simulink model "AdaptiveControlsProjectPart2_Sethi"  (R2019b)
settings: Solver=ode45  StartTime=0.0  StopTime=40  RelTol=1e-6
undefined symbols (not defined in the file): Ar, Astar, B, Br, Bstar, cur0, Gam, Gam_r, Gam_x, J, K, L, Lambda, lambda_star, linp, om0, P, phi0, Q, R, theta0, Tr_star, Tx_star, V0, w10, w20, Xr0
libraries: simulink x1
settings Model: Creator=aleon  LastModifiedBy=Japnit Sethi
settings SFSimCC: CustomCodeUndefinedFunction=UseInterfaceOnly

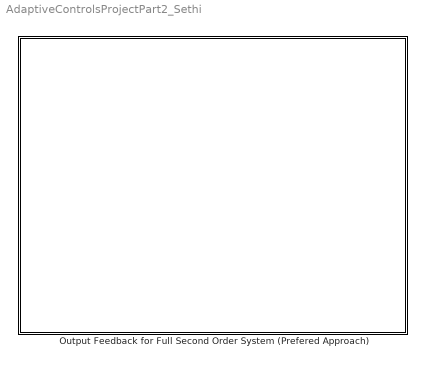
== system AdaptiveControlsProjectPart2_Sethi ==
  Output Feedback for Full Second Order System (Prefered Approach) : Subsystem

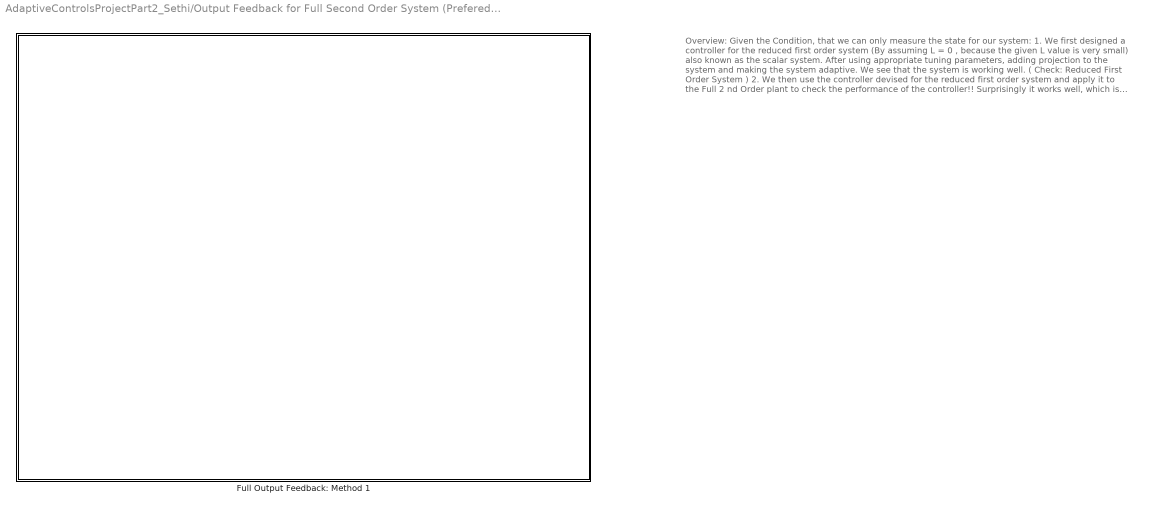
== system AdaptiveControlsProjectPart2_Sethi/Output Feedback for Full Second Order System (Prefered Approach) ==
  note: Overview:
      | Given the Condition, that we can only measure the state for our system:
      | 1. We first designed a controller for the reduced first order system (By assuming L = 0 , because the given L value is very small) also known as the scalar system. After using appropriate tuning parameters, adding projection to the system and making the system adaptive. We see that the system is working well. ( Check: Reduced First Order System )
      | 2. We then use the controller devised for the reduced first order system and apply it to the Full 2 nd Order plant to check the performance of the controller!! Surprisingly it works well, which is because the approximation of L was legible.
      | 3. We designed a Full state feedback controller for the Full second order system, by deriving the equations in canonical form and also change our states from and to and which is important in order to derive and satisfy our compatibility equations. In this scenario, we were able to measure both and . ( Check: Full Second Order System )
      | 4. Finally, we designed a Full Output Feedback controller , because in really, we cannot measure , the only measurement available to us is .
      | Note: ( Option 2: But not recommended ) For the Full output feedback controller above, we could measure and then calculate the by computing a numerical derivative of measured and adding a filter transfer function to get rid of the noise. But this is not preferred because excessive time that we can lose tuning our parameters to get rid of high oscillations and noise.
  Full Output Feedback: Method 1 : Subsystem

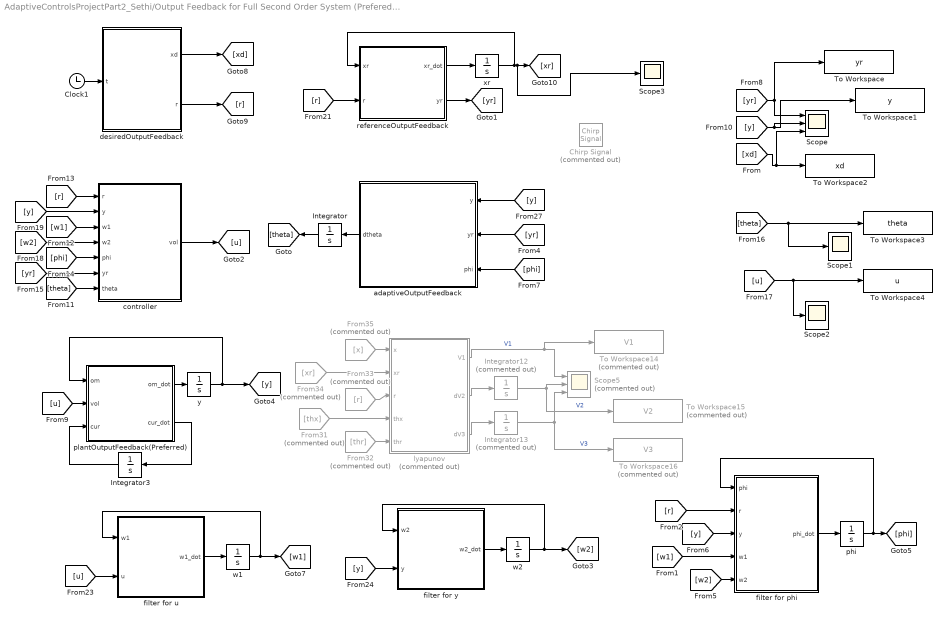
== system AdaptiveControlsProjectPart2_Sethi/Output Feedback for Full Second Order System (Prefered Approach)/Full Output Feedback: Method 1 ==
  Chirp Signal : simulink/Sources/Chirp Signal  Commented=on  f1=0.1  T=100  f2=1
  Clock1 : Clock
  From31 : From  Commented=on  GotoTag=thx
  From32 : From  Commented=on  GotoTag=thr
  From33 : From  Commented=on  GotoTag=r
  From34 : From  Commented=on  GotoTag=xr
  From35 : From  Commented=on  GotoTag=x
  Integrator : Integrator  InitialCondition=theta0
  Integrator12 : Integrator  Commented=on  InitialCondition=V0
  Integrator13 : Integrator  Commented=on  InitialCondition=V0
  Integrator3 : Integrator  InitialCondition=cur0
  Scope : Scope  NumInputPorts=3
  Scope1 : Scope
  Scope2 : Scope
  Scope3 : Scope
  Scope5 : Scope  Commented=on  NumInputPorts=3
  To Workspace : ToWorkspace  VariableName=yr  SampleTime=-1
  To Workspace1 : ToWorkspace  VariableName=y  SampleTime=-1
  To Workspace14 : ToWorkspace  Commented=on  VariableName=V1  SampleTime=-1
  To Workspace15 : ToWorkspace  Commented=on  VariableName=V2  SampleTime=-1
  To Workspace16 : ToWorkspace  Commented=on  VariableName=V3  SampleTime=-1
  To Workspace2 : ToWorkspace  VariableName=xd  SampleTime=-1
  To Workspace3 : ToWorkspace  VariableName=theta  SampleTime=-1
  To Workspace4 : ToWorkspace  VariableName=u  SampleTime=-1
  adaptiveOutputFeedback : MATLAB Function  TreatAsAtomicUnit=on
  controller : MATLAB Function  TreatAsAtomicUnit=on
  desiredOutputFeedback : MATLAB Function  TreatAsAtomicUnit=on
  filter for phi : MATLAB Function  TreatAsAtomicUnit=on
  filter for u : MATLAB Function  TreatAsAtomicUnit=on
  filter for y : MATLAB Function  TreatAsAtomicUnit=on
  lyapunov : MATLAB Function  Commented=on  TreatAsAtomicUnit=on
  phi : Integrator  InitialCondition=phi0
  plantOutputFeedback(Preferred) : MATLAB Function  TreatAsAtomicUnit=on
  referenceOutputFeedback : MATLAB Function  TreatAsAtomicUnit=on
  w1 : Integrator  InitialCondition=w10
  w2 : Integrator  InitialCondition=w20
  xr : Integrator  InitialCondition=Xr0
  y : Integrator  InitialCondition=om0
  wires:
  controller/1(vol) -> [u]
  [phi] -> adaptiveOutputFeedback/3(phi)
  xr/1 -> referenceOutputFeedback/1(xr), Scope3/1, [xr]
  [yr] -> Scope/1, To Workspace/1
  [w1] -> controller/3(w1)
  Clock1/1 -> desiredOutputFeedback/1(t)
  desiredOutputFeedback/2(r) -> [r]
  lyapunov/3(dV3) -> Integrator13/1
  Integrator3/1 -> plantOutputFeedback(Preferred)/3(cur)
  From31/1 -> lyapunov/4(thx)
  [y] -> filter for y/2(y)
  w1/1 -> [w1], filter for u/1(w1)
  Integrator13/1 -> Scope5/3, To Workspace16/1  "V3"
  lyapunov/2(dV2) -> Integrator12/1
  [w2] -> controller/4(w2)
  referenceOutputFeedback/1(xr_dot) -> xr/1
  y/1 -> [y], plantOutputFeedback(Preferred)/1(om)
  From35/1 -> lyapunov/1(x)
  lyapunov/1(V1) -> To Workspace14/1, Scope5/1  "V1"
  Integrator12/1 -> Scope5/2, To Workspace15/1  "V2"
  [phi] -> controller/5(phi)
  [u] -> To Workspace4/1, Scope2/1
  From33/1 -> lyapunov/3(r)
  [theta] -> Scope1/1, To Workspace3/1
  Integrator/1 -> [theta]
  [yr] -> adaptiveOutputFeedback/2(yr)
  From34/1 -> lyapunov/2(xr)
  filter for y/1(w2_dot) -> w2/1
  [xd] -> Scope/3, To Workspace2/1
  [r] -> controller/1(r)
  [y] -> To Workspace1/1, Scope/2
  w2/1 -> filter for y/1(w2), [w2]
  filter for u/1(w1_dot) -> w1/1
  [u] -> plantOutputFeedback(Preferred)/2(vol)
  plantOutputFeedback(Preferred)/2(cur_dot) -> Integrator3/1
  [r] -> referenceOutputFeedback/2(r)
  desiredOutputFeedback/1(xd) -> [xd]
  [y] -> adaptiveOutputFeedback/1(y)
  From32/1 -> lyapunov/5(thr)
  plantOutputFeedback(Preferred)/1(om_dot) -> y/1
  [u] -> filter for u/2(u)
  referenceOutputFeedback/2(yr) -> [yr]
  adaptiveOutputFeedback/1(dtheta) -> Integrator/1
  [theta] -> controller/7(theta)
  [y] -> controller/2(y)
  [yr] -> controller/6(yr)
  [r] -> filter for phi/2(r)
  [y] -> filter for phi/3(y)
  phi/1 -> filter for phi/1(phi), [phi]
  [w2] -> filter for phi/5(w2)
  [w1] -> filter for phi/4(w1)
  filter for phi/1(phi_dot) -> phi/1

== matlab function AdaptiveControlsProjectPart2_Sethi/Output Feedback for Full Second Order System (Prefered Approach)/Full Output Feedback: Method 1/filter for u ==
  data: w1 input; u input; w1_dot output; linp parameter; Lambda parameter
function w1_dot = filter_for_u(w1,u,linp, Lambda)

w1_dot = Lambda*w1 + linp*u; % linp is linput
% w1 is our filter for u

== matlab function AdaptiveControlsProjectPart2_Sethi/Output Feedback for Full Second Order System (Prefered Approach)/Full Output Feedback: Method 1/adaptiveOutputFeedback ==
  data: y input; yr input; phi input; dtheta output; Gam parameter; lambda_star parameter
function dtheta = adaptive(y,yr,phi,Gam, lambda_star)

e = y - yr;

dtheta = -(Gam*phi)*e*sign(lambda_star);

%%%%%%%%%%%%%%%%%%%%%%%%%%%%%%%%%%%%%%%%%%%
%------ Projection Algorithm Stuff  -----%
%%%%%%%%%%%%%%%%%%%%%%%%%%%%%%%%%%%%%%%%%%%
% theta = [thx; thr];
% dtheta = [dthx; dthr];
% 
% % Smooth Convex Function Pg. 121 "Adaptive Control Notes"
% convF = (theta'*theta - th_max^2)/(eps_th*th_max^2);
% 
% gradf = 2*theta/(eps_th*th_max^2);
% gradf_norm = gradf/norm(gradf); % Normalized Gradient (Eq. 203)Pg. 121 "Adaptive Control Notes"
% 
% % Note: vel is theta_dot
% vel_norm = dtheta'*gradf_norm;  % This is before saturation
% vel_norm2 = vel_norm; % 
% 
% % If I am outside the region
% if convF>0 && vel_norm>0   
%    new_dtheta = dtheta - gradf_norm*vel_norm*convF; % 3rd part of Eq. (203) Pg. 121 "Adaptive Control Notes"
%    dthx = new_dtheta(1:2);
%    dthr = new_dtheta(3);
%    vel_norm2 = new_dtheta'*gradf_norm; % Computed New velocity normal to compare with vel_norm !! Just to see how effective the algorithm was
%    % Don't really need vel_norm2, just for comparison purpose
%    % vel_norm2 is after SATURATION
% end

== matlab function AdaptiveControlsProjectPart2_Sethi/Output Feedback for Full Second Order System (Prefered Approach)/Full Output Feedback: Method 1/filter for phi ==
  data: phi input; r input; y input; phi_dot output; w1 input; w2 input; p0 parameter
%%%%%%%%%%%%%%%%%%%%%%%%%%%%%%%%%%%%%%%%%%%%%%%%
%------ Method 1: Taking the system as is -----%
%%%%%%%%%%%%%%%%%%%%%%%%%%%%%%%%%%%%%%%%%%%%%%%%

function phi_dot = filter_for_phi(phi,r,y,w1,w2,p0)

phi_dot = -p0*phi + [r ;  w1 ; y ; w2];

== matlab function AdaptiveControlsProjectPart2_Sethi/Output Feedback for Full Second Order System (Prefered Approach)/Full Output Feedback: Method 1/desiredOutputFeedback ==
  data: xd output; t input; r output; Ar parameter; Br parameter
function [xd,r] = desiredSecondOrder(t,Ar, Br)
xd = 10*sin(2*t);
dxd = 20*cos(2*t);
ddxd = -40*sin(2*t);

% r = (ddxd - ar1*xd - ar2*dxd)/br;
r = (ddxd - Ar(2,1)*xd - Ar(2,2)*dxd)/Br(2,1);

== matlab function AdaptiveControlsProjectPart2_Sethi/Output Feedback for Full Second Order System (Prefered Approach)/Full Output Feedback: Method 1/lyapunov ==
  data: x input; xr input; r input; V1 output; thx input; thr input; dV2 output; dV3 output; P parameter; Q parameter; Gam_x parameter; Gam_r parameter; Astar parameter; Br parameter; Tx_star parameter; Tr_star parameter; Bstar parameter; Ar parameter
function [V1,dV2,dV3] = lyapunov(x,xr,r,thx,thr,P,Q,Gam_x,Gam_r,...
                                 Astar,Br,Tx_star, Tr_star, Bstar, Ar)

P2 = P(:,2);

e = x - xr;
dV3= -e'*Q*e;

dthx = -Gam_x*(e'*P2)*x*sign(Bstar(2,1)); % -Gam_x*(e'*P2)*x*sign(bstar);
dthr = -Gam_r*(e'*P2)*r*sign(Bstar(2,1)); % -gam_r*(e'*P2)*r*sign(bstar);

vol = thx'*x + thr*r;
 
xr_dot = Ar*xr + Br*r;    % Ar*xr + [0 ; br]*r; 
x_dot = Astar*x + Bstar*vol; % [0 1;astar1 astar2]*x + [0 ; bstar]*vol;
edot= x_dot - xr_dot;

V1 = e'*P*e + abs(Bstar(2,1))*(thx - Tx_star)'*inv(Gam_x)*(thx - Tx_star) + ...
              abs(Bstar(2,1))/Gam_r*(thr - Tr_star)^2;
dV2 = edot'*P*e + e'*P*edot + 2*abs(Bstar(2,1))*(thx - Tx_star)'*inv(Gam_x)*dthx + ...
                              2*abs(Bstar(2,1))/Gam_r*(thr - Tr_star)*dthr;

== matlab function AdaptiveControlsProjectPart2_Sethi/Output Feedback for Full Second Order System (Prefered Approach)/Full Output Feedback: Method 1/controller ==
  data: r input; y input; w1 input; w2 input; phi input; vol output; yr input; lambda_star parameter; theta input; Gam parameter
%%%%%%%%%%%%%%%%%%%%%%%%%%%%%%%%%%%%%%%%%%%%%%%%
%------ Method 1: Taking the system as is -----%
%%%%%%%%%%%%%%%%%%%%%%%%%%%%%%%%%%%%%%%%%%%%%%%%

function vol = controller(r,y,w1,w2,phi,yr,lambda_star, theta, Gam)

e = y - yr;

vol = theta'*[r ;  w1 ; y ; w2] - phi'*Gam*phi*e*sign(lambda_star);
% phi is the additional pole

== matlab function AdaptiveControlsProjectPart2_Sethi/Output Feedback for Full Second Order System (Prefered Approach)/Full Output Feedback: Method 1/referenceOutputFeedback ==
  data: xr input; xr_dot output; r input; Ar parameter; Br parameter; yr output
function [xr_dot, yr] = referenceSecondOrder(xr, r, Ar, Br)

% xr_dot = [0, 1; ar1, ar2]*xr + [0; br]*r;
xr_dot = Ar*xr + Br*r;
yr = [1 0]*xr;

== matlab function AdaptiveControlsProjectPart2_Sethi/Output Feedback for Full Second Order System (Prefered Approach)/Full Output Feedback: Method 1/filter for y ==
  data: w2 input; y input; w2_dot output; linp parameter; Lambda parameter
function w2_dot = filter_for_y(w2,y,linp, Lambda)

w2_dot = Lambda*w2 + linp*y;
% w2 is our filter for y

== matlab function AdaptiveControlsProjectPart2_Sethi/Output Feedback for Full Second Order System (Prefered Approach)/Full Output Feedback: Method 1/plantOutputFeedback(Preferred) ==
  data: om input; om_dot output; vol input; cur input; J parameter; cur_dot output; L parameter; B parameter; K parameter; R parameter
function [om_dot,cur_dot] = plant(om,vol,cur, J, L, B, K, R)

om_dot = 1/J*(-B*om + K*cur);
cur_dot = 1/L*(-K*om - R*cur + vol);
